simulink model "sim_seq_example"  (Simulink 8.1)
settings: Solver=FixedStepDiscrete  StartTime=0.0  StopTime=5.0  FixedStep=1  RelTol=1e-3
libraries: simulink x4
settings Model: Creator=gcampa  LastModifiedBy=gcampa
settings DataIOCC: SignalLoggingSaveFormat=Dataset
settings OptimizationCC: ExpressionDepthLimit=128
settings DebuggingCC: FcnCallInpInsideContextMsg=EnableAllAsError
settings GRTTargetCC: CombineOutputUpdateFcns=on  GRTInterface=off

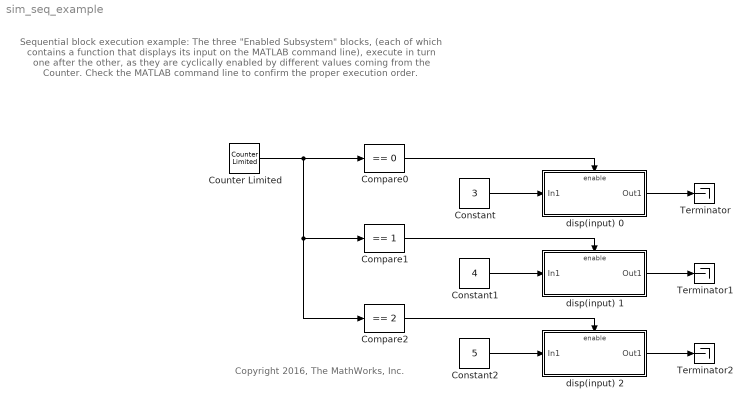
== system sim_seq_example ==
  note: Sequential block execution example:
      |
      | The three "Enabled Subsystem" blocks, (each of which contains a function that displays
      | its input on the MATLAB command line), execute in turn one after the other, as they are
      | cyclically enabled by different values coming from the Counter.
      |
      | Check the MATLAB command line to confirm the proper execution order.
  note: Copyright 2016, The MathWorks, Inc.
  Compare0 : simulink/Logic and Bit Operations/Compare To Constant  relop===  const=0  OutDataTypeStr=uint8
  Compare1 : simulink/Logic and Bit Operations/Compare To Constant  relop===  const=1  OutDataTypeStr=uint8
  Compare2 : simulink/Logic and Bit Operations/Compare To Constant  relop===  const=2  OutDataTypeStr=uint8
  Constant : Constant  Value=3
  Constant1 : Constant  Value=4
  Constant2 : Constant  Value=5
  Counter Limited : simulink/Sources/Counter Limited  uplimit=2  tsamp=-1
  Terminator : Terminator
  Terminator1 : Terminator
  Terminator2 : Terminator
  disp(input) 0 : Subsystem  TreatAsAtomicUnit=on
  disp(input) 1 : Subsystem  TreatAsAtomicUnit=on
  disp(input) 2 : Subsystem  TreatAsAtomicUnit=on
  wires:
  Constant/1 -> disp(input) 0/1(In1)
  Constant1/1 -> disp(input) 1/1(In1)
  disp(input) 0/1(Out1) -> Terminator/1
  disp(input) 1/1(Out1) -> Terminator1/1
  Constant2/1 -> disp(input) 2/1(In1)
  disp(input) 2/1(Out1) -> Terminator2/1
  Counter Limited/1 -> Compare2/1, Compare1/1, Compare0/1
  Compare0/1 -> disp(input) 0/Enable
  Compare1/1 -> disp(input) 1/Enable
  Compare2/1 -> disp(input) 2/Enable

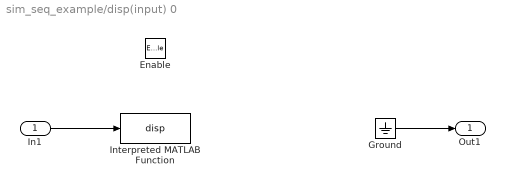
== system sim_seq_example/disp(input) 0 ==
  In1 : Inport
  Enable : EnablePort
  Ground : Ground
  Interpreted MATLAB Function : MATLABFcn  MATLABFcn=disp  OutputDimensions=0
  Out1 : Outport
  wires:
  In1/1 -> Interpreted MATLAB Function/1
  Ground/1 -> Out1/1

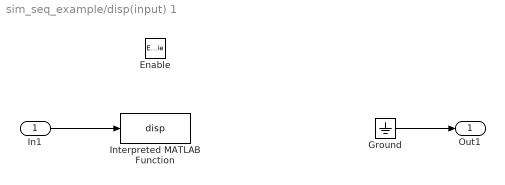
== system sim_seq_example/disp(input) 1 ==
  In1 : Inport
  Enable : EnablePort
  Ground : Ground
  Interpreted MATLAB Function : MATLABFcn  MATLABFcn=disp  OutputDimensions=0
  Out1 : Outport
  wires:
  Ground/1 -> Out1/1
  In1/1 -> Interpreted MATLAB Function/1

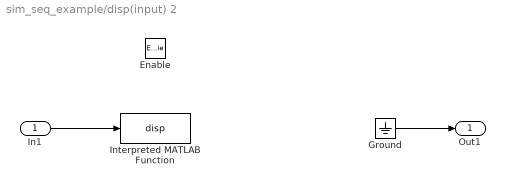
== system sim_seq_example/disp(input) 2 ==
  In1 : Inport
  Enable : EnablePort
  Ground : Ground
  Interpreted MATLAB Function : MATLABFcn  MATLABFcn=disp  OutputDimensions=0
  Out1 : Outport
  wires:
  In1/1 -> Interpreted MATLAB Function/1
  Ground/1 -> Out1/1
